simulink model "chris_1R_setpoint_og"  (R2016b)
settings: Solver=FixedStepDiscrete  StartTime=0.0  StopTime=5  FixedStep=0.1  MaxStep=0.1  RelTol=1e-3
libraries: realtime_pacer_lib x1, simulink x1
settings Model: Creator=RSL  LastModifiedBy=RSL

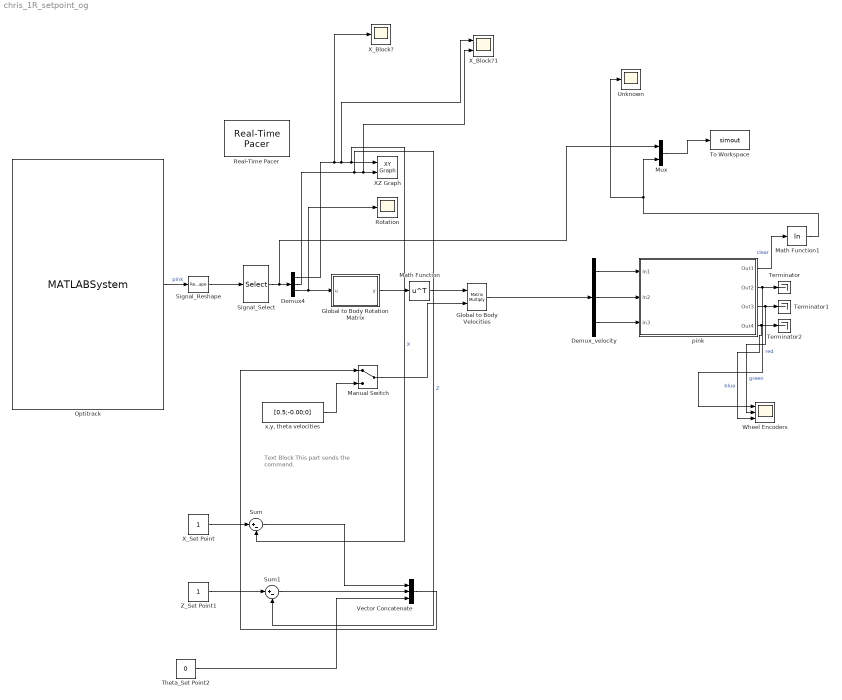
== system chris_1R_setpoint_og ==
  note: Text Block
      | This part sends the command.
  Demux4 : Demux  Outputs=3
  Demux_velocity : Demux  Outputs=3
  Global to Body Velocities : Product  Multiplication=Matrix(*)
  Global to Body Rotation Matrix : MATLAB Function  TreatAsAtomicUnit=on
  Manual Switch : ManualSwitch
  Math Function : Math  Operator=transpose  SaturateOnIntegerOverflow=on
  Math Function1 : Math  Operator=log  SaturateOnIntegerOverflow=on
  Mux : Mux  Inputs=2
  Optitrack : MATLABSystem  System=OptiTrackRigidBody  coordinateTransformationMatrix=[ 1, 0, 0; 0, 0, 1; 0, -1, 0 ]  rigidBodyNames={ 'pink'}  orientationFormat=Euler angles  debug=on  natNetHostAddress=127.0.0.1  natNetClientAddress=127.0.0.1  dllPath=C:\DecaMATLAB\NatNetSDK\lib\x64\NatNetML.dll  unicast=off
      mask Type: OptiTrackRigidBody
      mask Display:
      | disp('OptiTrackRigidBody');
      | port_label('output',1,'pink');
  Real-Time Pacer : realtime_pacer_lib/Real-Time Pacer  simTimePerRealTime=1
  Rotation : Scope
  Signal_Reshape : Reshape  OutputDimensions=6
  Signal_Select : Selector  InputPortWidth=6  IndexOptions=Index vector (dialog)  Indices=[1 2 6]  OutputSizes=1
  Sum : Sum  Inputs=|+-
  Sum1 : Sum  Inputs=|+-
  Terminator : Terminator
  Terminator1 : Terminator
  Terminator2 : Terminator
  Theta_Set Point2 : Constant  Value=0
  To Workspace : ToWorkspace  VariableName=simout  SaveFormat=Timeseries  SampleTime=-1
  Unknown : Scope
  Vector Concatenate : Concatenate  NumInputs=3
  "Wheel Encoders " : Scope  NumInputPorts=3
  XZ Graph : simulink/Sinks/XY Graph  xmin=-1  xmax=10  ymin=-1  ymax=10  st=-1
  X_Block? : Scope
  X_Block?1 : Scope  NumInputPorts=2
  X_Set Point : Constant
  Z_Set Point1 : Constant
  pink : Subsystem  mask(DecabotMask){robotName=pink, decabotHelper=localhost, robotAddress=, useDataTurbine=off, useDirectSocket=on, debug=off}
      mask prompts: robotName "Robot name:"; decabotHelper "DecabotHelper/DataTurbine server:"; robotAddress "Robot network address (optional):"; useDataTurbine "Use DataTurbine"; useDirectSocket "Use direct robot TCP connection"; debug "Log debug messages"
      mask help: This is a masked subsystem that contains a Decabot block for bidirectional communication with a decabot over a direct TCP socket connection.
      mask init:
      | robotName = 'Nobody';
      | decabotHelper = 'localhost';
      | robotAddress = '';
      | useDataTurbine = true;
      | debug = true;
      mask TypeOptions robotName: decabot/robotName
      mask Callback robotName:
      | try
      |     set_param( gcb( ), 'Name', get_param( gcb( ), 'robotName' ) );
      | end
      mask TypeOptions decabotHelper: decabot/decabotHelper
      mask TypeOptions robotAddress: decabot/robotAddress
      mask TypeOptions useDataTurbine: decabot/useDataTurbine
      mask TypeOptions useDirectSocket: decabot/useDirectSocket
      mask TypeOptions debug: decabot/debug
      mask Display:
      | disp( [get_param( gcb( ), 'robotName' ) '\n\nDH: ' get_param( gcb( ), 'decabotHelper' ) ] );
      | 
      | port_label('input',1,'x_vel');
      | port_label('input',2,'y_vel');
      | port_label('input',3,'t_vel');
      | 
      | port_label('output',1,'clear');
      | port_label('output',2,'red');
      | port_label('output',3,'green');
      | port_label('output',4,'blue');
  "x,y, theta velocities" : Constant  Value=[0.5;-0.00;0]
  wires:
  Optitrack/1 -> Signal_Reshape/1  "pink"
  Signal_Reshape/1 -> Signal_Select/1
  Global to Body Velocities/1 -> Demux_velocity/1
  Global to Body Rotation Matrix/1(y) -> Math Function/1
  Signal_Select/1 -> Mux/1, Demux4/1
  Math Function/1 -> Global to Body Velocities/1
  Demux_velocity/3 -> pink/3(In3)
  Demux_velocity/1 -> pink/1(In1)
  Demux_velocity/2 -> pink/2(In2)
  pink/2(Out2) -> "Wheel Encoders "/1, Terminator/1  "red"
  pink/3(Out3) -> "Wheel Encoders "/2, Terminator1/1  "green"
  pink/4(Out4) -> "Wheel Encoders "/3, Terminator2/1  "blue"
  pink/1(Out1) -> Math Function1/1  "clear"
  Demux4/3 -> Rotation/1, Global to Body Rotation Matrix/1(u)
  Demux4/1 -> X_Block?/1, X_Block?1/1, Sum/2, XZ Graph/1  "X"
  Demux4/2 -> Sum1/2, X_Block?1/2, XZ Graph/2  "Z"
  "x,y, theta velocities"/1 -> Manual Switch/2
  Manual Switch/1 -> Global to Body Velocities/2
  Math Function1/1 -> Unknown/1, Mux/2
  Mux/1 -> To Workspace/1
  Sum/1 -> Vector Concatenate/1
  Vector Concatenate/1 -> Manual Switch/1
  X_Set Point/1 -> Sum/1
  Z_Set Point1/1 -> Sum1/1
  Sum1/1 -> Vector Concatenate/2
  Theta_Set Point2/1 -> Vector Concatenate/3

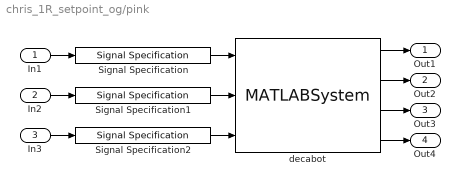
== system chris_1R_setpoint_og/pink ==
  In1 : Inport
  In2 : Inport  Port=2
  In3 : Inport  Port=3
  Signal Specification : SignalSpecification  OutDataTypeStr=double  Dimensions=1
  Signal Specification1 : SignalSpecification  OutDataTypeStr=double  Dimensions=1
  Signal Specification2 : SignalSpecification  OutDataTypeStr=double  Dimensions=1
  decabot : MATLABSystem  System=Decabot  robotName=pink  decabotHelper=localhost  useDataTurbine=off  useDirectSocket=on  debug=off
      mask Type: Decabot
      mask Display:
      | disp('pink\n\nDH: localhost');
      | port_label('input',1,'x_vel');
      | port_label('input',2,'y_vel');
      | port_label('input',3,'t_vel');
      | port_label('output',1,'clear');
      | port_label('output',2,'red');
      | port_label('output',3,'green');
      | port_label('output',4,'blue');
  Out1 : Outport
  Out2 : Outport  Port=2
  Out3 : Outport  Port=3
  Out4 : Outport  Port=4
  wires:
  Signal Specification2/1 -> decabot/3
  Signal Specification1/1 -> decabot/2
  Signal Specification/1 -> decabot/1
  In2/1 -> Signal Specification1/1
  decabot/4 -> Out4/1
  decabot/1 -> Out1/1
  decabot/3 -> Out3/1
  decabot/2 -> Out2/1
  In1/1 -> Signal Specification/1
  In3/1 -> Signal Specification2/1

== matlab function chris_1R_setpoint_og/Global to Body Rotation Matrix ==
  data: u input; y output
function y = fcn(u)

y = [cos(u) -sin(u) 0; sin(u) cos(u) 0; 0 0 1];
